simulink model "Q2"  (R2020b)
settings: Solver=VariableStepAuto  StartTime=0.0  StopTime=10.0  RelTol=1e-3
settings Model: Creator=asus  LastModifiedBy=asus

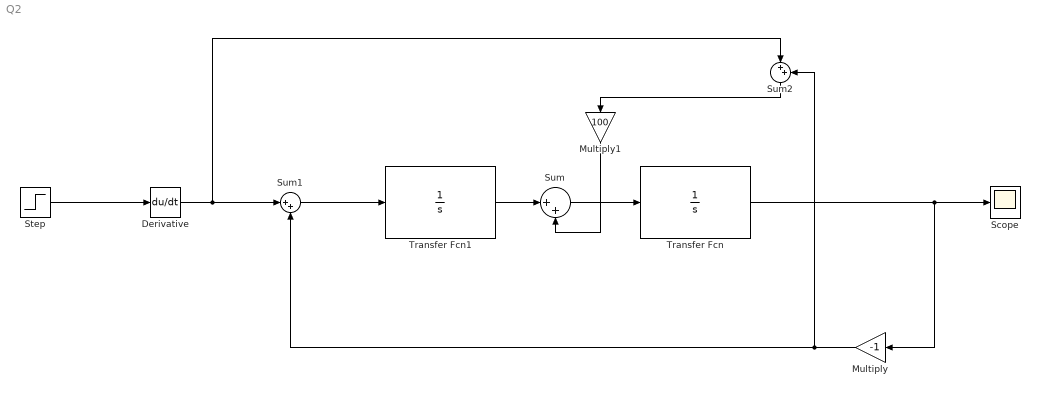
== system Q2 ==
  Derivative : Derivative
  Multiply : Gain  Gain=-1
  Multiply1 : Gain  Gain=100
  Scope : Scope
  Step : Step  Time=0.001  SampleTime=0
  Sum : Sum  Inputs=|++
  Sum1 : Sum  Inputs=|++
  Sum2 : Sum  Inputs=|++
  Transfer Fcn : TransferFcn  Denominator=[1 0]
  Transfer Fcn1 : TransferFcn  Denominator=[1 0]
  wires:
  Transfer Fcn/1 -> Multiply/1, Scope/1
  Sum1/1 -> Transfer Fcn1/1
  Multiply/1 -> Sum1/2, Sum2/2
  Sum2/1 -> Multiply1/1
  Step/1 -> Derivative/1
  Derivative/1 -> Sum2/1, Sum1/1
  Multiply1/1 -> Sum/2
  Sum/1 -> Transfer Fcn/1
  Transfer Fcn1/1 -> Sum/1
